simulink model "sldemo_hydrod"  (R2022b)
settings: Solver=ode45  StartTime=0.0  StopTime=0.1  RelTol=1e-3  AbsTol=1e-6
model workspace (MATLAB code in the model file):
  | % Load the initial conditions and initialization data
  | % Using the same MAT file as
  | % sldemo_hydcyl
  | % sldemo_hydcyl4
  | % sldemo_hydrod
  | 
  | load sldemo_hydcyl_data;
undefined symbols (not defined in the file or in its folder): Ac, C2, I, L, M, Qmax
libraries: hydlib x4, simulink x2
(part 2 of 2)

== system sldemo_hydrod/More Info ==

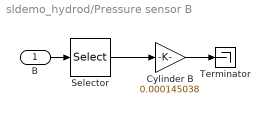
== system sldemo_hydrod/Pressure sensor B ==
  B : Inport
  Cylinder B : Gain  Gain=0.000145038
  Selector : Selector  InputPortWidth=2  IndexOptions=Index vector (dialog)  Indices=1  OutputSizes=1
  Terminator : Terminator
  wires:
  B/1 -> Selector/1
  Selector/1 -> Cylinder B/1
  Cylinder B/1 -> Terminator/1

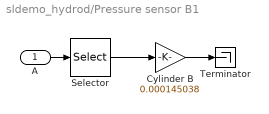
== system sldemo_hydrod/Pressure sensor B1 ==
  A : Inport
  Cylinder B : Gain  Gain=0.000145038
  Selector : Selector  InputPortWidth=2  IndexOptions=Index vector (dialog)  Indices=1  OutputSizes=1
  Terminator : Terminator
  wires:
  Cylinder B/1 -> Terminator/1
  Selector/1 -> Cylinder B/1
  A/1 -> Selector/1
